simulink model "step3"  (R2026a)
settings: Solver=VariableStepAuto  StopTime=30
undefined symbols (not defined in the file or in its folder): A, Cd, F_drive, m, rho, theta
settings Model: Creator=manoj  LastModifiedBy=manoj

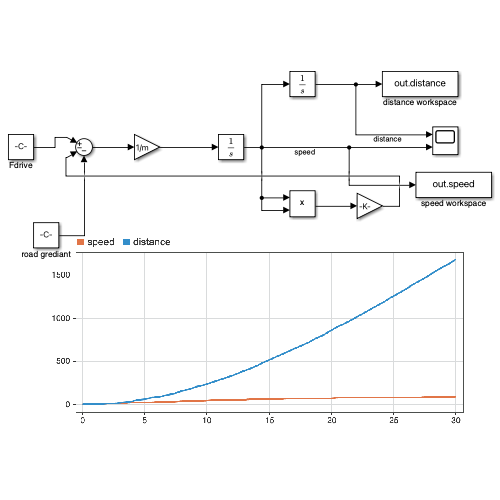
[thumbnail: Simulink's stored preview of the top-level diagram]
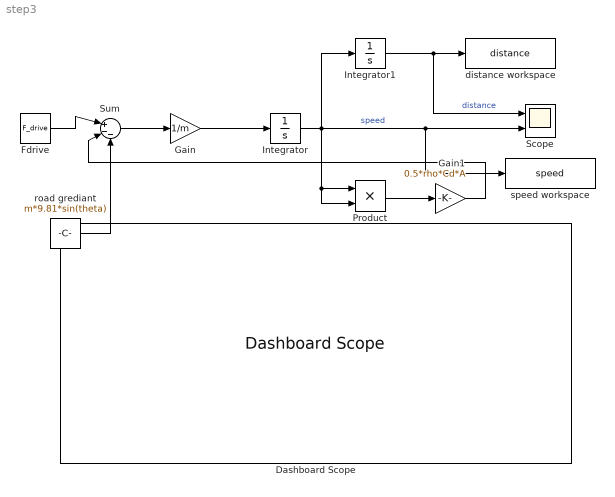
== system step3 ==
  Dashboard Scope : DashboardScope  FontColor=[0.0, 0.0, 0.0]
  Fdrive : Constant  Value=F_drive
  Gain : Gain  Gain=1/m
  Gain1 : Gain  Gain=0.5*rho*Cd*A
  Integrator : Integrator
  Integrator1 : Integrator
  Product : Product
  Scope : Scope  NumInputPorts=2
      settings: ActiveDisplayYMinimum=-1  ActiveDisplayYMaximum=1
  Sum : Sum  Inputs=|+--
  distance workspace : ToWorkspace  VariableName=distance  SaveFormat=Structure With Time  SampleTime=-1
  road grediant : Constant  Value=m*9.81*sin(theta)
  speed workspace : ToWorkspace  VariableName=speed  SaveFormat=Structure With Time  SampleTime=-1
  wires:
  Fdrive/1 -> Sum/1
  Sum/1 -> Gain/1
  Gain/1 -> Integrator/1
  Integrator/1 -> Product/2, Product/1, Integrator1/1, speed workspace/1, Scope/2  "speed"
  Integrator1/1 -> distance workspace/1, Scope/1  "distance"
  Product/1 -> Gain1/1
  Gain1/1 -> Sum/2
  road grediant/1 -> Sum/3
